simulink model "C172_Plant"  (R2025a)
settings: Solver=ode4  StartTime=startTime  StopTime=stopTime  FixedStep=stepTime  RelTol=1e-3
values from neighbouring files (symbols this model uses):
  C172MasterModel =     [C172MasterModel.mat]
undefined symbols (not defined in the file or in its folder): ft, kg, m, slug
libraries: aerolibconvert2 x2, aerolib6dof2 x1, matrix_library x1, aerolibatmos2 x1, aerolibasang x1
settings Model: Creator=avi  LastModifiedBy=avi
settings DataIOCC: ExternalInput=RPM, df_deg, da_rad, de_rad, dr_rad  LoadExternalInput=on  SaveFormat=StructureWithTime

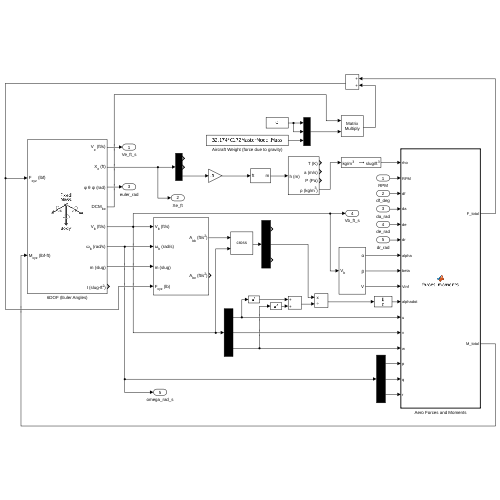
[thumbnail: Simulink's stored preview of the top-level diagram]
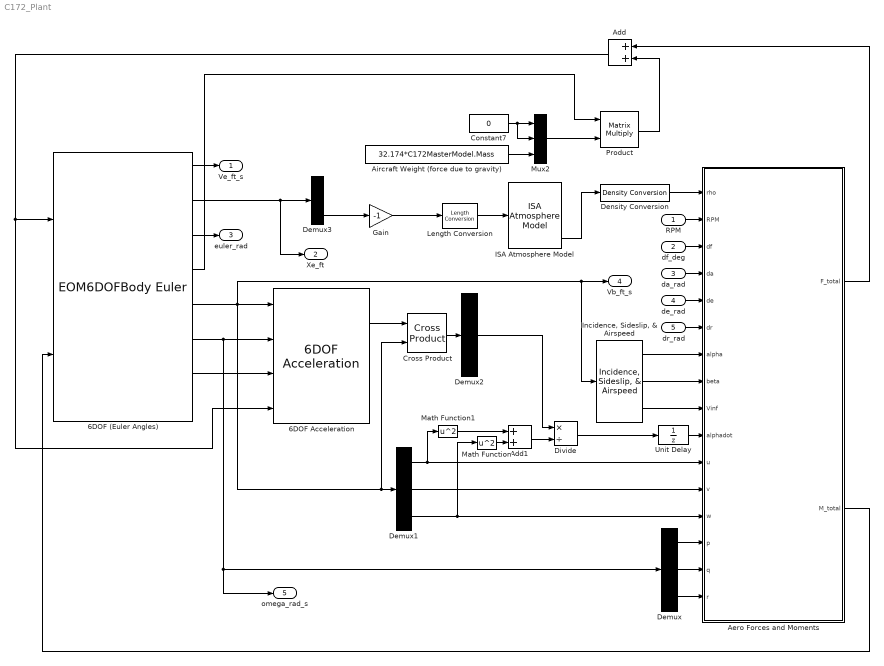
== system C172_Plant ==
  RPM : Inport
  df_deg : Inport  Port=2
  da_rad : Inport  Port=3
  de_rad : Inport  Port=4
  dr_rad : Inport  Port=5
  6DOF (Euler Angles) : EOM6DOFBodyEuler  units=English (velocity in ft/s)  xme_0=Pos0  Vm_0=Vel0  eul_0=Att0  pm_0=Ome0  mass_0=C172MasterModel.Mass  inertia=C172MasterModel.Inertia  mass_flag=on
  6DOF Acceleration : aerolib6dof2/6DOF Acceleration  units=English (Velocity in ft/s)  mtype=Fixed  vre_flag=off
  Add : Sum
  Add1 : Sum
  Aero Forces and Moments : MATLAB Function  TreatAsAtomicUnit=on
  Aircraft Weight (force due to gravity) : Constant  Value=32.174*C172MasterModel.Mass
  Constant7 : Constant  Value=0
  Cross Product : matrix_library/Cross Product
  Demux{,1..3} (4 alike) : Demux  Outputs=3
  Density Conversion : aerolibconvert2/Density Conversion  IU=kg/m^3  OU=slug/ft^3
  Divide : Product  Inputs=*/
  Gain : Gain  Gain=-1
  ISA Atmosphere Model : aerolibatmos2/ISA Atmosphere Model  useExtended=off  action=None  custom=off  viscosityOut=off  g=9.80665  gamma=1.4  R=287.0531  L=0.0065  h_trop=11000  h_strat=20000  rho0=1.225  P0=101325  T0=288.15  h0=0  S=110.4  Tref=273.15  muref=1.716e-5
  "Incidence, Sideslip, & Airspeed" : aerolibasang/Incidence, Sideslip, & Airspeed
  Length Conversion : aerolibconvert2/Length Conversion  IU=ft  OU=m
  Math Function : Math  Operator=square
  Math Function1 : Math  Operator=square
  Mux2 : Mux  Inputs=3
  Product : Product  Multiplication=Matrix(*)
  Unit Delay : UnitDelay  SampleTime=-1  HasFrameUpgradeWarning=on
  Ve_ft_s : Outport
  Xe_ft : Outport  Port=2
  euler_rad : Outport  Port=3
  Vb_ft_s : Outport  Port=4
  omega_rad_s : Outport  Port=5
  wires:
  6DOF (Euler Angles)/5 -> "Incidence, Sideslip, & Airspeed"/1, Vb_ft_s/1, 6DOF Acceleration/1, Demux1/1, Cross Product/2
  df_deg/1 -> Aero Forces and Moments/3(df)
  da_rad/1 -> Aero Forces and Moments/4(da)
  de_rad/1 -> Aero Forces and Moments/5(de)
  dr_rad/1 -> Aero Forces and Moments/6(dr)
  "Incidence, Sideslip, & Airspeed"/1 -> Aero Forces and Moments/7(alpha)
  "Incidence, Sideslip, & Airspeed"/2 -> Aero Forces and Moments/8(beta)
  Demux/3 -> Aero Forces and Moments/16(r)
  6DOF (Euler Angles)/6 -> 6DOF Acceleration/2, omega_rad_s/1, Demux/1
  Demux/1 -> Aero Forces and Moments/14(p)
  Demux/2 -> Aero Forces and Moments/15(q)
  Aero Forces and Moments/2(M_total) -> 6DOF (Euler Angles)/2
  Constant7/1 -> Mux2/1, Mux2/2
  Aircraft Weight (force due to gravity)/1 -> Mux2/3
  6DOF (Euler Angles)/4 -> Product/1
  Mux2/1 -> Product/2
  Product/1 -> Add/2
  Add/1 -> 6DOF (Euler Angles)/1, 6DOF Acceleration/4
  Aero Forces and Moments/1(F_total) -> Add/1
  6DOF (Euler Angles)/2 -> Demux3/1, Xe_ft/1
  6DOF (Euler Angles)/1 -> Ve_ft_s/1
  6DOF (Euler Angles)/3 -> euler_rad/1
  "Incidence, Sideslip, & Airspeed"/3 -> Aero Forces and Moments/9(Vinf)
  Demux1/3 -> Math Function/1, Aero Forces and Moments/13(w)
  Demux1/1 -> Math Function1/1, Aero Forces and Moments/11(u)
  RPM/1 -> Aero Forces and Moments/2(RPM)
  6DOF (Euler Angles)/7 -> 6DOF Acceleration/3
  6DOF Acceleration/1 -> Cross Product/1
  Cross Product/1 -> Demux2/1
  Demux2/2 -> Divide/1
  Demux1/2 -> Aero Forces and Moments/12(v)
  Add1/1 -> Divide/2
  Divide/1 -> Unit Delay/1
  Math Function1/1 -> Add1/1
  Math Function/1 -> Add1/2
  Unit Delay/1 -> Aero Forces and Moments/10(alphadot)
  Length Conversion/1 -> ISA Atmosphere Model/1
  Demux3/3 -> Gain/1
  Density Conversion/1 -> Aero Forces and Moments/1(rho)
  ISA Atmosphere Model/4 -> Density Conversion/1
  Gain/1 -> Length Conversion/1

== matlab function C172_Plant/Aero Forces and Moments ==
  data: rho input; F_total output size=[3,1]; M_total output size=[3,1]; RPM input; df input; da input; de input; dr input; alpha input; beta input; Vinf input; alphadot input; u input; v input; w input; p input; q input; r input; C172MasterModel parameter
function [F_total, M_total] = forces_moments(rho, RPM, df, da, de, dr, alpha, beta, Vinf, alphadot, u, v, w, p, q, r, C172MasterModel)

%% Load constant parameters from the C172 Master Model
Sw = C172MasterModel.Sw;
Cbar = C172MasterModel.Cbar;
bw = C172MasterModel.bw;
CG = C172MasterModel.CG;
D = C172MasterModel.D;
Kp = C172MasterModel.Kp;
PropIxx = C172MasterModel.PropIxx;
AeroRP = C172MasterModel.AeroRP;
Engine = C172MasterModel.Engine;

qbar = (0.5)*rho*Vinf^2;

%% Engine Calculations
Va = u - (q*(Engine(3) - CG(3))) - (r*(Engine(2) - CG(2))); % q term is negative to account for structural to FRD frame conversion

n = RPM/60;
J = Va/(n*D);

T = rho*(n^2)*(D^4)*interp1(C172MasterModel.Tables.CT.RowBP, C172MasterModel.Tables.CT.Data, J);
Q = rho*(n^2)*(D^5)*(1/(2*pi))*(-1)*interp1(C172MasterModel.Tables.CP.RowBP, C172MasterModel.Tables.CP.Data, J);

if isnan(T)
    error('Simulation halted: CT lookup out of bounds. Input was %f.', J);
end
if isnan(Q)
    error('Simulation halted: CP lookup out of bounds. Input was %f.', J);
end


% Map Structural Coordinates to Body Frame Moment Arms
% Structural: +X aft, +Y right, +Z up
% Body:       +X fwd, +Y right, +Z down
dy_struct = Engine(2) - CG(2);
dz_struct = Engine(3) - CG(3);
ry = dy_struct;
rz = -dz_struct;

Np = (-1)*T*Kp*D*alpha;
Ml = T*rz;
Nl = (-1)*T*ry;

Mg = (-1)*PropIxx*2*pi*n*r;
Ng = PropIxx*2*pi*n*q;

F_thrust = [T; 0; 0];
M_thrust = [Q; (Ml + Mg); (Np + Nl + Ng)];

A = pi*((D/2)^2);
Vpw = (0.5)*((-1)*Va + sqrt(Va^2 + ((2*T)/(rho*A))));
qbar_pw = (0.5)*rho*Vpw^2;

Vinduced = u + Vpw;
qbar_induced = (0.5)*rho*Vinduced^2;


%% Aero Forces

% Calculate all the drag force components
CDo = qbar*Sw*0.027;
CDDf = qbar*Sw*interp1(C172MasterModel.Tables.CDDf.RowBP, C172MasterModel.Tables.CDDf.Data, df);
CDwbh = qbar*Sw*interp2(C172MasterModel.Tables.CDwbh.ColBP, C172MasterModel.Tables.CDwbh.RowBP, C172MasterModel.Tables.CDwbh.Data, df, alpha);
CDbeta = qbar*Sw*norm(beta)*0.15;
% Calculate total drag force
Drag = CDo + CDDf + CDwbh + CDbeta;

if isnan(CDDf)
    error('Simulation halted: CDDf lookup out of bounds. Input was %f.', df);
end
if isnan(CDwbh)
    error('Simulation halted: CDwbh lookup out of bounds. Input was %f and %f.', df, alpha);
end

% Calculate all the side force components
CYb = qbar*Sw*interp2(C172MasterModel.Tables.CYb.ColBP, C172MasterModel.Tables.CYb.RowBP, C172MasterModel.Tables.CYb.Data, df, beta);
CYdr = qbar*Sw*dr*0.15;
% Calculate total side force
Side = CYb + CYdr;

if isnan(CYb)
    error('Simulation halted: CYb lookup out of bounds. Input was %f and %f.', df, beta);
end

% Calculate all the lift force components
CLwbh = qbar*Sw*interp1(C172MasterModel.Tables.CLwbh.RowBP, C172MasterModel.Tables.CLwbh.Data, alpha);
CLDf = qbar*Sw*interp1(C172MasterModel.Tables.CLDf.RowBP, C172MasterModel.Tables.CLDf.Data, df);
CLDe = qbar*Sw*de*0.43;
CLadot = qbar*Sw*alphadot*(Cbar/(2*Vinf))*1.7;
CLq = qbar*Sw*q*(Cbar/(2*Vinf))*3.9;
% Calculate total lift force
Lift = CLwbh + CLDf + CLDe + CLadot + CLq;

if isnan(CLwbh)
    error('Simulation halted: CLwbh lookup out of bounds. Input was %f.', alpha);
end
if isnan(CLDf)
    error('Simulation halted: CLDf lookup out of bounds. Input was %f.', df);
end


%% Aero Moments

% Calculate roll moment components
Clb = qbar*Sw*bw*beta*(-0.092);
Clp = qbar*Sw*bw*(bw/(2*Vinf))*p*(-0.484);
Clr = qbar*Sw*bw*(bw/(2*Vinf))*r*interp1(C172MasterModel.Tables.Clr.RowBP, C172MasterModel.Tables.Clr.Data, alpha);
ClDa = qbar*Sw*bw*da*0.2;
Cldr = qbar*Sw*bw*dr*0.0147;
% Calculate total roll moment
Roll = Clb + Clp + Clr + ClDa + Cldr;

if isnan(Clr)
    error('Simulation halted: Clr lookup out of bounds. Input was %f.', alpha);
end


% Calculate pitch moment components
Cmo = qbar*Sw*Cbar*interp1(C172MasterModel.Tables.Cmo.RowBP, C172MasterModel.Tables.Cmo.Data, qbar);
Cmalpha = qbar*Sw*Cbar*alpha*(-1);
Cmq = qbar*Sw*Cbar*(Cbar/(2*Vinf))*q*(-12.4);
Cmadot = qbar*Sw*Cbar*(Cbar/(2*Vinf))*alphadot*(-7.27);
Cmde = qbar_induced*Sw*Cbar*de*(-1);
Cmdf = qbar*Sw*Cbar*interp1(C172MasterModel.Tables.Cmdf.RowBP, C172MasterModel.Tables.Cmdf.Data, df);
% Calculate total pitch moment
Pitch = Cmo + Cmalpha + Cmq + Cmadot + Cmde + Cmdf;

if isnan(Cmo)
    error('Simulation halted: Cmo lookup out of bounds. Input was %f.', qbar);
end
if isnan(Cmdf)
    error('Simulation halted: Cmdf lookup out of bounds. Input was %f.', df);
end


% Calculate yaw moment components
Cnb = qbar*Sw*bw*interp1(C172MasterModel.Tables.Cnb.RowBP, C172MasterModel.Tables.Cnb.Data, beta);
Cnspw = qbar_pw*Sw*bw*(-0.05);
Cnr = qbar*Sw*bw*(bw/(2*Vinf))*r*(-0.0937);
Cnda = qbar*Sw*bw*da*interp2(C172MasterModel.Tables.Cnda.ColBP, C172MasterModel.Tables.Cnda.RowBP, C172MasterModel.Tables.Cnda.Data, beta, alpha);
Cnp = qbar*Sw*bw*(bw/(2*Vinf))*p*interp1(C172MasterModel.Tables.Cnp.RowBP, C172MasterModel.Tables.Cnp.Data, alpha);
Cndr = qbar_induced*Sw*bw*dr*(-0.0645);
% Calculate total yaw moment
Yaw = Cnb + Cnspw + Cnr + Cnda + Cnp + Cndr;

if isnan(Cnb)
    error('Simulation halted: Cnb lookup out of bounds. Input was %f.', beta);
end
if isnan(Cnda)
    error('Simulation halted: Cnda lookup out of bounds. Input was %f and %f.', beta, alpha);
end
if isnan(Cnp)
    error('Simulation halted: Cnp lookup out of bounds. Input was %f.', alpha);
end


%% Transform Aero Forces to Body Axes
% Lift and Drag rotated by alpha. Sideforce is already in Body Y.
F_Ax = -Drag * cos(alpha) + Lift * sin(alpha);
F_Ay = Side;
F_Az = -Drag * sin(alpha) - Lift * cos(alpha);

F_aero = [F_Ax; F_Ay; F_Az];

%% Map Structural Coordinates to Body Frame Moment Arms
% Structural: +X aft, +Y right, +Z up
% Body:       +X fwd, +Y right, +Z down
dx_struct = AeroRP(1) - CG(1);
dy_struct = AeroRP(2) - CG(2);
dz_struct = AeroRP(3) - CG(3);

rx = -dx_struct;
ry = dy_struct;
rz = -dz_struct;

%% Calculate Induced Moments at CG (Cross Product: r x F)
delta_Roll  = (ry * F_Az) - (rz * F_Ay);
delta_Pitch = (rz * F_Ax) - (rx * F_Az);
delta_Yaw   = (rx * F_Ay) - (ry * F_Ax);

%% Sum Total Aero Moments in Body Axes
M_Total_Roll  = Roll + delta_Roll;
M_Total_Pitch = Pitch + delta_Pitch;
M_Total_Yaw   = Yaw + delta_Yaw;

M_aero = [M_Total_Roll; M_Total_Pitch; M_Total_Yaw];


%% Final sum of forces and moments
F_total = F_aero + F_thrust;
M_total = M_aero + M_thrust;

end
